simulink model "ControleFF_D_NL"  (R2020b)
settings: Solver=ode23  StartTime=0  StopTime=11  FixedStep=rate  RelTol=1e-3
values from neighbouring files (symbols this model uses):
  Beff = 50    [controle_FF.m]    (also in controle_PD.m)
  Jeff = 0.5    [controle_FF.m]    (also in controle_PD.m)
  K = (90/12)*(2*pi/60)    (= 0.785398163397)    [controle_FF.m]    (also in controle_PD.m)
  Kd = (2*xi*wn*Jeff - Beff)/K    (= -44.5633840657)    [controle_FF.m]    (also in controle_PD.m)
  Kp = (wn^2*Jeff)/K    (= 143.239448783)    [controle_FF.m]    (also in controle_PD.m)
  N = 3    [controle_FF.m]    (also in controle_PD.m)
  r = 1./[231.22*4 139.138 139.138 231.22 231.22]    [controle_FF.m]    (also in controle_PD.m)
undefined symbols (not defined in the file or in its folder): alpha, Fc, Fs, phi
libraries: simulink_extras x7
(part 5 of 5)

== matlab function ControleFF_D_NL/Compensador Feedforward/Perturbação_d/MATLAB Function3 ==
  data: M input; V input; tau1 output; G input; ddTh input
function tau1  = calcul_dk1(M, V, G, ddTh)

tau1 = M(1,2)*ddTh(2) + M(1,3)*ddTh(3) + M(1,4)*ddTh(4) + M(1,5)*ddTh(5) ...
       + V(1) + G(1);
